simulink model "Mass_est"  (R2023b)
settings: Solver=VariableStepAuto  StartTime=T_start  StopTime=T_stop  FixedStep=T_step  RelTol=1e-3
undefined symbols (not defined in the file): Aux_power, Batt_mdens, Battmassfrac, Crr, fwdorbwd, g, lengths, Mass, roadcurvatures, V_end, V_start
libraries: autolibshared x2, drivinglib x1
settings Model: Creator=cas  LastModifiedBy=cas
settings DataIOCC: ExternalInput=150  ReturnWorkspaceOutputs=off  LoggingToFile=on
settings OptimizationCC: ZeroExternalMemoryAtStartup=off  ZeroInternalMemoryAtStartup=off
settings RTWCC: TargetLang=C++
settings GRTTargetCC: TargetLangStandard=C++11 (ISO)  CodeInterfacePackaging=C++ class

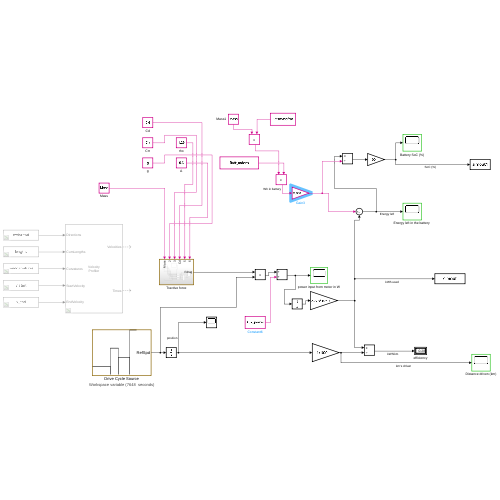
[thumbnail: Simulink's stored preview of the top-level diagram]
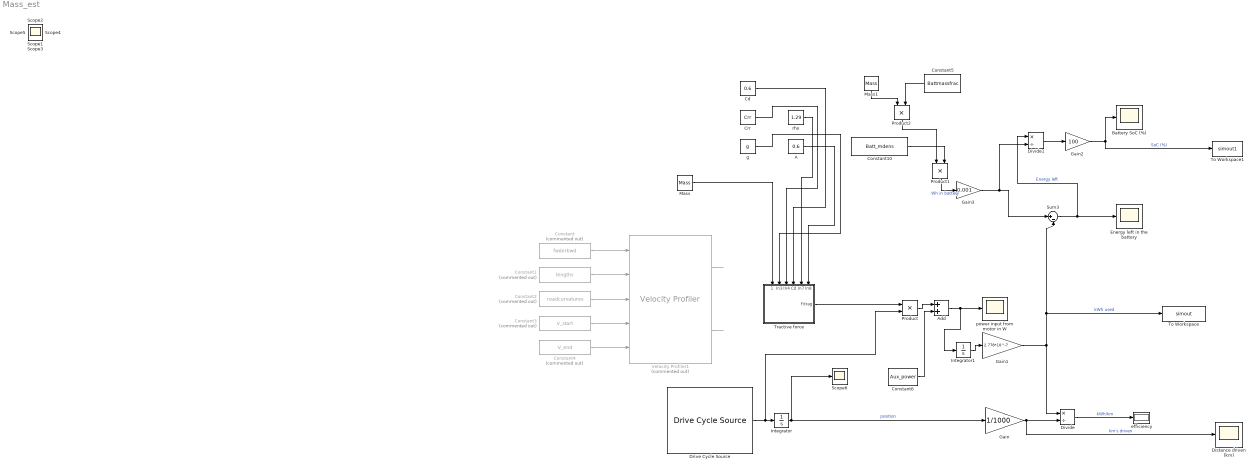
== system Mass_est ==
  A : Constant  Value=0.6
  Add : Sum
  Battery SoC (%) : Scope
  Cd : Constant  Value=0.6
  Constant : Constant  Commented=on  Value=fwdorbwd
  Constant1 : Constant  Commented=on  Value=lengths
  Constant10 : Constant  Value=Batt_mdens
  Constant2 : Constant  Commented=on  Value=roadcurvatures
  Constant3 : Constant  Commented=on  Value=V_start
  Constant4 : Constant  Commented=on  Value=V_end
  Constant5 : Constant  Value=Battmassfrac
  Constant6 : Constant  Value=Aux_power
  Crr : Constant  Value=Crr
  Distance driven (km) : Scope
  Divide : Product  Inputs=*/
  Divide1 : Product  Inputs=*/
  Drive Cycle Source : autolibshared/Drive Cycle Source  cycleVar=Workspace variable  wsVar=velocity_profile  fileVar=cycleFTP75.mat  tfinal="7648  seconds"  cycleRepeat=off  outAccPort=off  outGearPort=off  gearList=No gear data  t_wot1=5  xdot_woto=0  xdot_wot1=30  t_wot2=20  xdot_wot2=0  t_wotend=30  srcUnit=km/h  outUnit=m/s  srcAccUnit=m/s/s  outAccUnit=m/s^2  dt=0  aMode=1  faultOption=off  velBnd=2  velBndUnit=mph  inUnit=m/s  timeBnd=1  failOption=off  stopSim=off  maxFaultCnt=10  maxFaultTime=2  maxTotFaultTime=15  traceOption=off  dtTrace=1  traceWindow=10  lastDCname=Custom Data Set  lastOutUnit=mph  lastDT=0  lastTB=1  lastSB=2  forceCalcBound=off
  "Energy left in the battery " : Scope
  Gain : Gain  Gain=1/1000
  Gain1 : Gain  Gain=2.778*10^-7
  Gain2 : Gain  Gain=100
  Gain3 : Gain  Gain=0.001
  Integrator : Integrator
  Integrator1 : Integrator
  Mass : Constant  Value=Mass
  Mass1 : Constant  Value=Mass
  Product : Product
  Product1 : Product
  Product2 : Product
  Scope{1..6} (6 alike) : Scope
  Sum3 : Sum  Inputs=|+-
  To Workspace : ToWorkspace  VariableName=simout  SampleTime=-1
      settings: Decimation=2  Save2DSignal=2-D array (concatenate along first dimension)
  To Workspace1 : ToWorkspace  VariableName=simout1  SampleTime=-1
      settings: Decimation=2  Save2DSignal=2-D array (concatenate along first dimension)
  Tractive force : Subsystem
      settings: PortSchema="{\"entries\":[{\"content\":{\"sides\":[{\"content\":{},\"type\":\"ConnectorPlacement.EquallySpacedRectSide\",\"uuid\":\"1dc941f5-3e74-4cbf-a52e-ea3cab36909e\"},{\"content\":{\"connectorIds\":[\"Out1\"],\"side\":\"RIGHT\"},\"type\":\"ConnectorPlacement.EquallySpacedRectSide\",\"uuid\":\"6f8e9dcb-b594-405f-a2b1-c41d344efafb\"},{\"content\":{\"connectorIds\":[\"In1\",\"In2\",\"In3\",\"In4\",\"In5\",\"In6\"],\"side\":\"TOP\"},\"type\":\"ConnectorPlacement.EquallySpacedRectSide\",\"uuid\":\"1ae95007-d3a7-4d64-89c5-5ad33b1ab93d\"}]},\"type\":\"ConnectorPlacement.EquallySpacedConnector\",\"uuid\":\"adcee74b-2e32-4cf6-bb91-c8e1408d67ea\"}],\"packageUris\":[\"http://schema.mathworks.com/mf0/Connector/R2020b\"],\"version\":\"1.0\"}"
  Velocity Profiler1 : drivinglib/Velocity Profiler  Commented=on  MaxLongitudinalAccel=3  MaxLongitudinalDecel=1  MaxSpeed=maxspeed  MaxLongitudinalJerk=1  MaxLateralAccel=1  ShowOptionalOutport=on  SampleTime=0.1  SimulateUsing=Code generation
  efficiency : Display
      settings: Format=bank
  g : Constant  Value=g
  power input from motor in W : Scope
  rho : Constant  Value=1.29
  wires:
  rho/1 -> Tractive force/5(In7)
  Constant3/1 -> Velocity Profiler1/4
  Constant/1 -> Velocity Profiler1/1
  Cd/1 -> Tractive force/4(Cd)
  Tractive force/1(Fdrag) -> Product/1
  g/1 -> Tractive force/2(In3)
  Constant4/1 -> Velocity Profiler1/5
  Mass/1 -> Tractive force/1(Mass)
  Velocity Profiler1/1 -> ?
  Velocity Profiler1/2 -> ?
  Integrator1/1 -> Gain1/1
  Constant1/1 -> Velocity Profiler1/2
  Divide/1 -> efficiency/1  "kWh/km"
  Gain1/1 -> Divide/1, To Workspace/1, Sum3/2  "kWh used"
  Crr/1 -> Tractive force/3(In4)
  A/1 -> Tractive force/6(In8)
  Product1/1 -> Gain3/1  "Wh in battery"
  Gain/1 -> Distance driven (km)/1, Divide/2  "km's driven"
  Constant2/1 -> Velocity Profiler1/3
  Integrator/1 -> Scope6/1, Gain/1  "position"
  Drive Cycle Source/1 -> Product/2, Integrator/1
  Constant10/1 -> Product1/2
  Sum3/1 -> Divide1/1, "Energy left in the battery "/1  "Energy left"
  Divide1/1 -> Gain2/1
  Gain2/1 -> To Workspace1/1, Battery SoC (%)/1  "SoC (%)"
  Product/1 -> Add/1
  Constant6/1 -> Add/2
  Add/1 -> Integrator1/1, power input from motor in W/1
  Mass1/1 -> Product2/1
  Constant5/1 -> Product2/2
  Product2/1 -> Product1/1
  Gain3/1 -> Divide1/2, Sum3/1

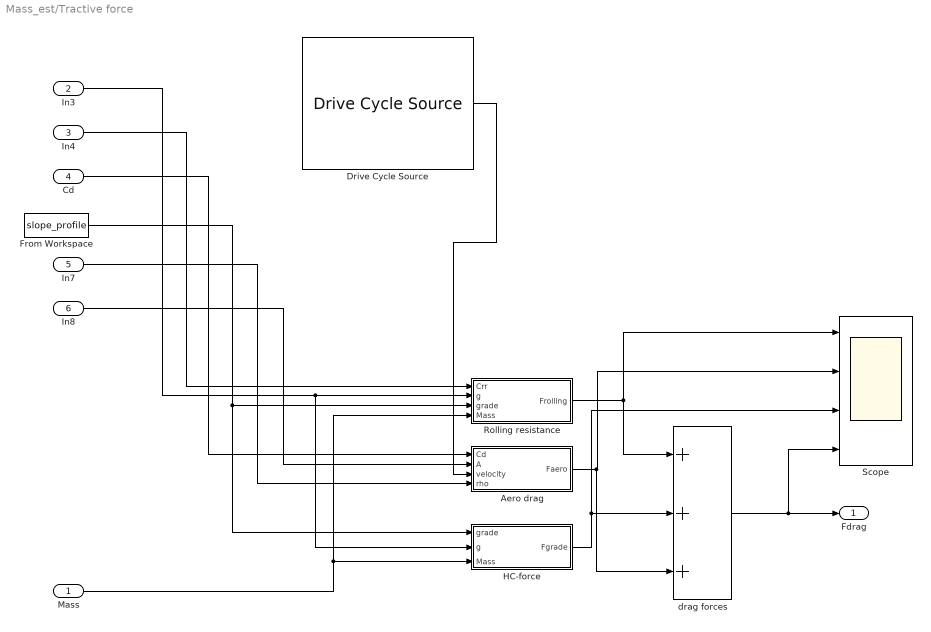
== system Mass_est/Tractive force ==
  Mass : Inport
  In3 : Inport  Port=2
  In4 : Inport  Port=3
  Cd : Inport  Port=4
  In7 : Inport  Port=5
  In8 : Inport  Port=6
  Aero drag : Subsystem
  Drive Cycle Source : autolibshared/Drive Cycle Source  cycleVar=Workspace variable  wsVar=velocity_profile  fileVar=cycleFTP75.mat  tfinal="7648  seconds"  cycleRepeat=off  outAccPort=off  outGearPort=off  gearList=No gear data  t_wot1=5  xdot_woto=0  xdot_wot1=30  t_wot2=20  xdot_wot2=0  t_wotend=30  srcUnit=km/h  outUnit=m/s  srcAccUnit=m/s/s  outAccUnit=m/s^2  dt=0  aMode=1  faultOption=off  velBnd=2  velBndUnit=mph  inUnit=m/s  timeBnd=1  failOption=off  stopSim=off  maxFaultCnt=10  maxFaultTime=2  maxTotFaultTime=15  traceOption=off  dtTrace=1  traceWindow=10  lastDCname=Custom Data Set  lastOutUnit=mph  lastDT=0  lastTB=1  lastSB=2  forceCalcBound=off
  From Workspace : FromWorkspace  VariableName=slope_profile
  HC-force : Subsystem
  Rolling resistance : Subsystem
  Scope : Scope  NumInputPorts=4
  drag forces : Sum  Inputs=+++
  Fdrag : Outport
  wires:
  Rolling resistance/1(Frolling) -> drag forces/1, Scope/1
  HC-force/1(Fgrade) -> Scope/3, drag forces/2
  drag forces/1 -> Scope/4, Fdrag/1
  Aero drag/1(Faero) -> drag forces/3, Scope/2
  Drive Cycle Source/1 -> Aero drag/3(velocity)
  Mass/1 -> Rolling resistance/4(Mass), HC-force/3(Mass)
  In3/1 -> HC-force/2(g), Rolling resistance/2(g)
  In4/1 -> Rolling resistance/1(Crr)
  Cd/1 -> Aero drag/1(Cd)
  From Workspace/1 -> HC-force/1(grade), Rolling resistance/3(grade)
  In7/1 -> Aero drag/4(rho)
  In8/1 -> Aero drag/2(A)

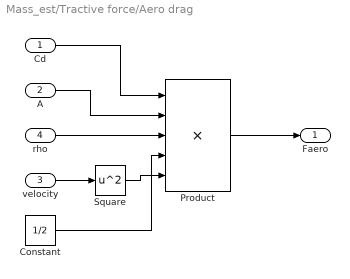
== system Mass_est/Tractive force/Aero drag ==
  Cd : Inport
  A : Inport  Port=2
  velocity : Inport  Port=3
  rho : Inport  Port=4
  Constant : Constant  Value=1/2
  Product : Product  Inputs=5
  Square : Math  Operator=square
  Faero : Outport
  wires:
  Cd/1 -> Product/1
  velocity/1 -> Square/1
  A/1 -> Product/2
  Square/1 -> Product/5
  Constant/1 -> Product/4
  Product/1 -> Faero/1
  rho/1 -> Product/3

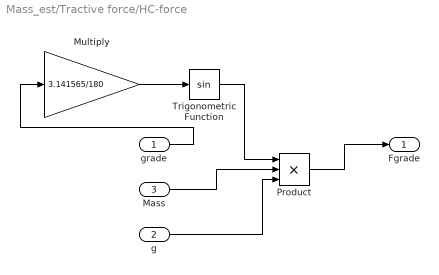
== system Mass_est/Tractive force/HC-force ==
  grade : Inport
  g : Inport  Port=2
  Mass : Inport  Port=3
  Multiply : Gain  Gain=3.141565/180
  Product : Product  Inputs=3
  Trigonometric Function : Trigonometry
  Fgrade : Outport
  wires:
  grade/1 -> Multiply/1
  Multiply/1 -> Trigonometric Function/1
  Trigonometric Function/1 -> Product/1
  Mass/1 -> Product/2
  g/1 -> Product/3
  Product/1 -> Fgrade/1

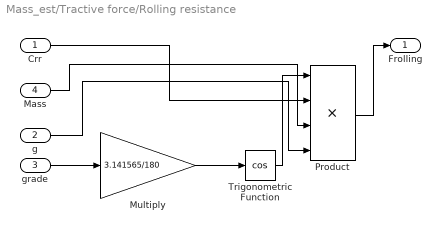
== system Mass_est/Tractive force/Rolling resistance ==
  Crr : Inport
  g : Inport  Port=2
  grade : Inport  Port=3
  Mass : Inport  Port=4
  Multiply : Gain  Gain=3.141565/180
  Product : Product  Inputs=4
  Trigonometric Function : Trigonometry  Operator=cos
  Frolling : Outport
  wires:
  Crr/1 -> Product/2
  Mass/1 -> Product/3
  g/1 -> Product/4
  grade/1 -> Multiply/1
  Multiply/1 -> Trigonometric Function/1
  Trigonometric Function/1 -> Product/1
  Product/1 -> Frolling/1
